simulink model "Open_loop"  (R2016b)
settings: Solver=VariableStepAuto  StartTime=0.0  StopTime=20  RelTol=1e-3
undefined symbols (not defined in the file or in its folder): A_lat, A_long, B_lat, B_long, C_lat, C_long, D_lat, D_long
libraries: dspsrcs4 x4
settings Model: Creator=yashm  LastModifiedBy=yashm

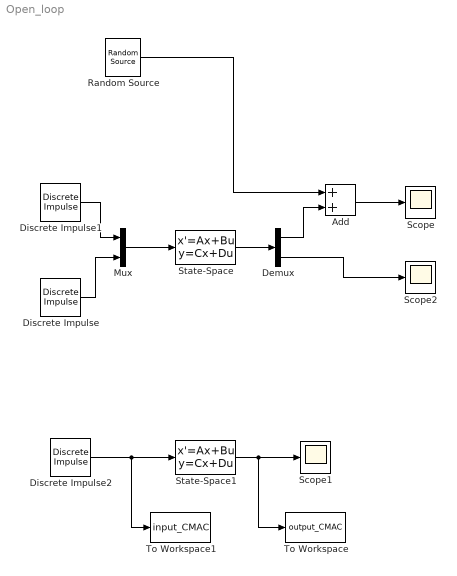
== system Open_loop ==
  Add : Sum
  Demux : Demux  Outputs=2
  Discrete Impulse : dspsrcs4/Discrete  Impulse  Delay=0  SampleTime=1  FrameSample=1  OutputFrames=off  dataType=double  isSigned=on  wordLen=16  udDataType=sfix(16)  fracBitsMode=Best precision  numFracBits=15  OutDataTypeStr=double  LastOutDataTypeStr=double
  Discrete Impulse1 : dspsrcs4/Discrete  Impulse  Delay=0  SampleTime=1  FrameSample=1  OutputFrames=off  dataType=double  isSigned=on  wordLen=16  udDataType=sfix(16)  fracBitsMode=Best precision  numFracBits=15  OutDataTypeStr=double  LastOutDataTypeStr=double
  Discrete Impulse2 : dspsrcs4/Discrete  Impulse  Delay=0  SampleTime=1  FrameSample=1  OutputFrames=off  dataType=double  isSigned=on  wordLen=16  udDataType=sfix(16)  fracBitsMode=Best precision  numFracBits=15  OutDataTypeStr=double  LastOutDataTypeStr=double
  Mux : Mux  Inputs=2
  Random Source : dspsrcs4/Random Source  SrcType=Uniform  NormMethod=Ziggurat  CltLength=12  MinVal=0  MaxVal=0.5  MeanVal=0  VarVal=1  RepMode=Not repeatable  rawSeed=1  IsInherit=off  SampMode=Discrete  SampTime=0.1  SampFrame=10  DataType=Double  OutComplex=Real  OutputFrames=off
  Scope : Scope
  Scope1 : Scope
  Scope2 : Scope
  State-Space : StateSpace  A=A_lat  B=B_lat  C=C_lat  D=D_lat  X0=0
  State-Space1 : StateSpace  A=A_long  B=B_long  C=C_long  D=D_long  X0=0
  To Workspace : ToWorkspace  VariableName=output_CMAC  SampleTime=-1
      settings: Save2DSignal=2-D array (concatenate along first dimension)
  To Workspace1 : ToWorkspace  VariableName=input_CMAC  SampleTime=-1
      settings: Save2DSignal=2-D array (concatenate along first dimension)
  wires:
  Demux/2 -> Scope2/1
  Mux/1 -> State-Space/1
  Discrete Impulse/1 -> Mux/2
  Discrete Impulse1/1 -> Mux/1
  State-Space1/1 -> To Workspace/1, Scope1/1
  Discrete Impulse2/1 -> To Workspace1/1, State-Space1/1
  Random Source/1 -> Add/1
  State-Space/1 -> Demux/1
  Add/1 -> Scope/1
  Demux/1 -> Add/2
